simulink model "Lab2_5"  (Simulink 7.3)
settings: Solver=ode45  StartTime=0.0  StopTime=0.3  RelTol=1e-3
libraries: simulink x2
settings Model: Creator=Seva  LastModifiedBy=Seva

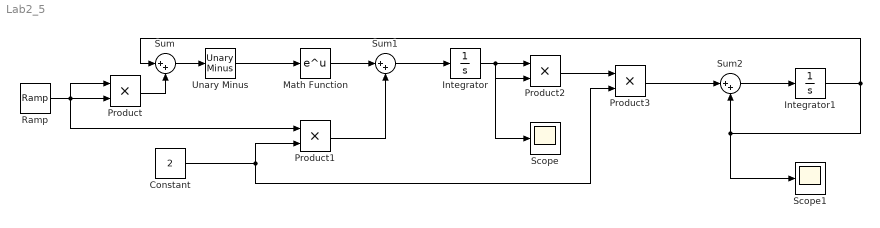
== system Lab2_5 ==
  Constant : Constant  Value=2  OutDataType=fixdt(1, 16)  OutScaling=2^0
  Integrator : Integrator  InitialCondition=0.5
  Integrator1 : Integrator  InitialCondition=1
  Math Function : Math  OutDataType=fixdt(1, 16)  OutScaling=2^0  SaturateOnIntegerOverflow=on
  Product{,1..3} (4 alike) : Product  OutDataType=fixdt(1, 16)  OutScaling=2^0  RndMeth=Zero
  Ramp : simulink/Sources/Ramp  SystemSampleTime=-1  slope=1  start=0  X0=0
  Scope : Scope
  Scope1 : Scope
  Sum : Sum  Inputs=|++  OutDataType=fixdt(1, 16)  OutScaling=2^0
  Sum1 : Sum  Inputs=|++  OutDataType=fixdt(1, 16)  OutScaling=2^0
  Sum2 : Sum  Inputs=|++  OutDataType=fixdt(1, 16)  OutScaling=2^0
  Unary Minus : simulink/Math Operations/Unary Minus  DoSatur=off
  wires:
  Ramp/1 -> Product/2, Product/1, Product1/1
  Product/1 -> Sum/2
  Sum/1 -> Unary Minus/1
  Unary Minus/1 -> Math Function/1
  Constant/1 -> Product1/2, Product3/2
  Math Function/1 -> Sum1/1
  Product1/1 -> Sum1/2
  Sum1/1 -> Integrator/1
  Integrator/1 -> Product2/1, Product2/2, Scope/1
  Product2/1 -> Product3/1
  Product3/1 -> Sum2/1
  Sum2/1 -> Integrator1/1
  Integrator1/1 -> Sum/1, Sum2/2, Scope1/1
